simulink model "power_xfosaturable"  (Simulink 6.0)
settings: Solver=ode15s  SolverMode=SingleTasking  StartTime=0.0  StopTime=0.5  RelTol=1e-3  AbsTol=1e-2
libraries: powerlib x10
settings Model: Creator=patrice  LastModifiedBy=batserve  ExtModeTrigMode=oneshot  ExtModeArmWhenConnect=off  ExtModeAutoUpdateStatusClock=off
settings DataIOCC: LimitDataPoints=off  SignalLoggingName=sigsOut
settings OptimizationCC: BlockReduction=off  BooleanDataType=off
settings DebuggingCC: SolverPrmCheckMsg=none  UnconnectedInputMsg=none  UnconnectedOutputMsg=none  UnconnectedLineMsg=none
settings HardwareCC: TargetUnknown=on
settings RTWCC: TemplateMakefile=grt_unix.tmf

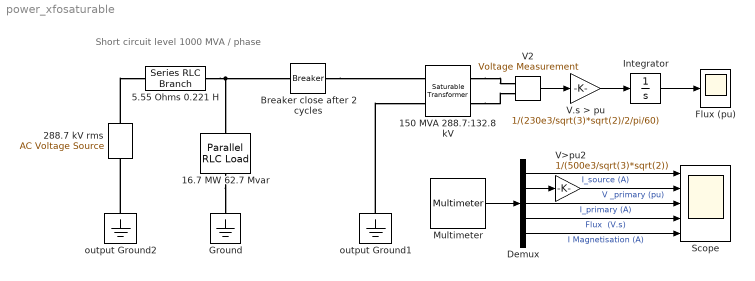
== system power_xfosaturable ==
  note: Short circuit level
      | 1000 MVA / phase
  150 MVA 288.7:132.8 kV : powerlib/Elements/Saturable Transformer  NominalPower=[ 150e6 60 ]  Winding1=[ 500e3/sqrt(3) 0.002 0.08 ]  Winding2=[ 230e3/sqrt(3) 0.002 0.08]  ThreeWindings=off  Winding3=[ 230e3/sqrt(3) 0.002 0.08]  Saturation="[0 0;  0.0 1.2; 1.0  1.52]"  CoreLoss=[500 0.8]  Hysteresis=off  DataFile='hysteresis_SI'  Measurements=All measurements (V I Flux)  InitialFlux=0  TransfoNumber=1
      settings: AttributesFormatString=\n
  16.7 MW 62.7 Mvar : powerlib/Elements/Parallel RLC Load  Orientation=down  PhysicalDomain=powersysdomain  SubClassName=unknown  LeftPortType=p1  RightPortType=p1  LConnTagsString=a  RConnTagsString=__new0  NominalVoltage=500e3/sqrt(3)  NominalFrequency=60  ActivePower=16.7e6  InductivePower=0  CapacitivePower=62.7e6  Measurements=None
      settings: AttributesFormatString=\n
  288.7 kV rms : powerlib/Electrical Sources/AC Voltage Source  Description=source block  Orientation=up  Amplitude=500e3/sqrt(3)*sqrt(2)  Phase=0  Frequency=60  SampleTime=0  Measurements=None
      settings: AttributesFormatString=\n
  "5.55 Ohms 0.221 H " : powerlib/Elements/Series RLC Branch  PhysicalDomain=powersysdomain  SubClassName=unknown  LeftPortType=p1  RightPortType=p1  LConnTagsString=__new0  RConnTagsString=__new0  Resistance=5.55  Inductance=0.221  Capacitance=inf  Measurements=Branch current
  Breaker close after 2 cycles : powerlib/Elements/Breaker  BreakerResistance=0.01  InitialState=0  SnubberResistance=100e6  SnubberCapacitance=inf  SwitchingTimes=[ 2/60 ]  External=off  Measurements=None
      settings: AttributesFormatString=\n
  Demux : Demux  Outputs=5
  Flux (pu) : Scope
      settings: DeleteFcn=simscope BlockIsBeingDestroyed  PostSaveFcn=simscope Save  TickLabels=on  TimeRange=0.5  YMin=-0.25  YMax=2.25  DataFormat=Array
  Ground : powerlib/Elements/Ground  Orientation=down  PhysicalDomain=powersysdomain  SubClassName=unknown  LeftPortType=p1  RightPortType=p1  LConnTagsString=a
  Integrator : Integrator  InitialCondition=0.8
  Multimeter : powerlib/Measurements/Multimeter  Tag=PoWeRsYsTeMmEaSuReMeNt  PhasorSimulation=off  OutputType=Magnitude  sel=[3 1 4 8 7]  L=8  Gain=[1 1 1 1 1]  yselected={'Ib: 5.55 Ohms 0.221 H ','Uw1: 150 MVA 288.7:132.8 kV','Iw1: 150 MVA 288.7:132.8 kV','Flux: 150 MVA 288.7:132.8 kV','Imag: 150 MVA 288.7:132.8 kV'};  PSBOutputType=1  PSBequivalent=0  AxesSetting=[0,0.1,-100,100]  Display=0  SavedBlockNames=-11
      settings: AttributesFormatString=\n
  Scope : Scope  NumInputPorts=5
      settings: DeleteFcn=simscope BlockIsBeingDestroyed  PostSaveFcn=simscope Save  TimeRange=0.5  YMin=-500~-1.5~-500~0~-500  YMax=2500~1.5~2500~2500~2500  SaveName=R
  V.s > pu : Gain  Gain=1/(230e3/sqrt(3)*sqrt(2)/2/pi/60)  SaturateOnIntegerOverflow=on
  V2 : powerlib/Measurements/Voltage Measurement  Tag=PoWeRsYsTeMmEaSuReMeNt  PhasorSimulation=off  OutputType=Magnitude  PSBequivalent=0
  V>pu2 : Gain  Gain=1/(500e3/sqrt(3)*sqrt(2))  SaturateOnIntegerOverflow=on
  output Ground1 : powerlib/Elements/Ground  Orientation=down  PhysicalDomain=powersysdomain  SubClassName=unknown  LeftPortType=p1  RightPortType=p1  LConnTagsString=a
  output Ground2 : powerlib/Elements/Ground  Orientation=down  PhysicalDomain=powersysdomain  SubClassName=unknown  LeftPortType=p1  RightPortType=p1  LConnTagsString=a
  wires:
  Integrator/1 -> Flux (pu)/1
  V.s > pu/1 -> Integrator/1
  Demux/1 -> Scope/1  "I_source (A)"
  Demux/3 -> Scope/3  "I_primary (A)"
  Demux/4 -> Scope/4  "Flux  (V.s)"
  Demux/2 -> V>pu2/1
  V>pu2/1 -> Scope/2  "V _primary (pu)"
  Demux/5 -> Scope/5  "I Magnetisation (A)"
  V2/1 -> V.s > pu/1
  Multimeter/1 -> Demux/1
  connections:
  288.7 kV rms/RConn1 -- "5.55 Ohms 0.221 H "/LConn1
  output Ground2/LConn1 -- 288.7 kV rms/LConn1
  "5.55 Ohms 0.221 H "/RConn1 -- 16.7 MW 62.7 Mvar/LConn1 -- Breaker close after 2 cycles/LConn1
  16.7 MW 62.7 Mvar/RConn1 -- Ground/LConn1
  output Ground1/LConn1 -- 150 MVA 288.7:132.8 kV/LConn2
  Breaker close after 2 cycles/RConn1 -- 150 MVA 288.7:132.8 kV/LConn1
  150 MVA 288.7:132.8 kV/RConn1 -- V2/LConn1
  150 MVA 288.7:132.8 kV/RConn2 -- V2/LConn2
